simulink model "Testbench"  (R2022b)
settings: Solver=ode1  StartTime=0.0  StopTime=10.0  FixedStep=0.1  RelTol=1e-3
PreLoadFcn:
  | run("Fzg_par.m")
values from neighbouring files (symbols this model uses):
  c_alpha_H = 13400    [Fzg_Par.m]    (also in Fzg_par.m)
  c_alpha_V = 9300    [Fzg_Par.m]    (also in Fzg_par.m)
  delta_H = 0    [Fzg_Par.m]    (also in Fzg_par.m)
  delta_V = delta_L/i_L    (= 1.01419878296)    [Fzg_Par.m]    (also in Fzg_par.m = -1.01419878296)
  l_fzg = 1300/1000    (= 1.3)    [Fzg_par.m]
  l_H_fzg = 507/1000    (= 0.507)    [Fzg_Par.m]    (also in Fzg_par.m)
  l_V_fzg = 1023/1000    (= 1.023)    [Fzg_Par.m]    (also in Fzg_par.m)
  m_fzg = 241.5 + 82    (= 323.5)    [Fzg_Par.m]    (also in Fzg_par.m)
  ss_A = [-(c_alpha_V*l_V_fzg^2+c_alpha_H*l_H_fzg^2)/(J_fzg_z*v_x) (c_alpha_H*l_H_fzg-c_alpha_V*l_V_fzg)/J_fzg_z ... (first row only)    [Fzg_par.m]
  ss_B = [(c_alpha_V*l_V_fzg)/J_fzg_z -(c_alpha_H*l_H_fzg)/J_fzg_z ... (first row only)    [Fzg_par.m]
  ss_C = [1 0]    [Fzg_par.m]
  ss_D = [0 0]    [Fzg_par.m]
  v_x = 15    [Fzg_Par.m]    (also in Fzg_par.m = 10)
settings Model: LastModifiedBy=timos
settings OptimizationCC: ReuseModelBlockBuffer=on
settings RTWCC: GPUComputeCapability=5.0
settings ConfigComp: CovBoundaryAbsTol=1.0e-5

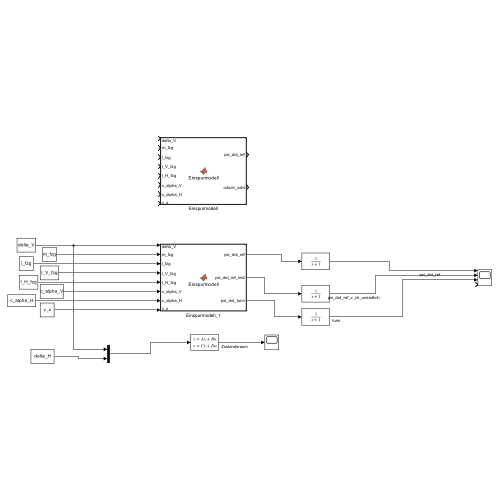
[thumbnail: Simulink's stored preview of the top-level diagram]
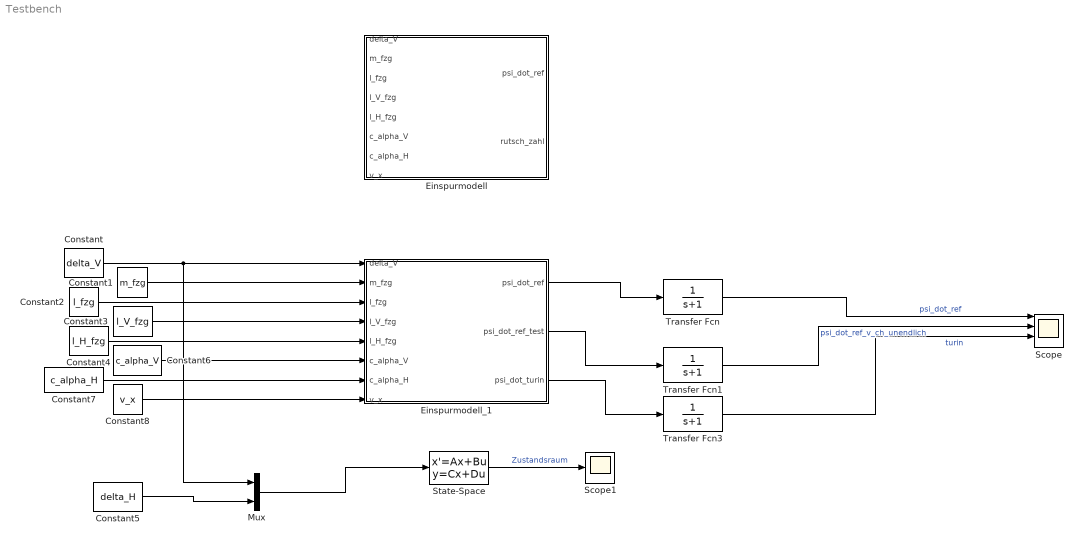
== system Testbench ==
  Constant : Constant  Value=delta_V
  Constant1 : Constant  Value=m_fzg
  Constant2 : Constant  Value=l_fzg
  Constant3 : Constant  Value=l_V_fzg
  Constant4 : Constant  Value=l_H_fzg
  Constant5 : Constant  Value=delta_H
  Constant6 : Constant  Value=c_alpha_V
  Constant7 : Constant  Value=c_alpha_H
  Constant8 : Constant  Value=v_x
  Einspurmodell : MATLAB Function  TreatAsAtomicUnit=on
  Einspurmodell_1 : MATLAB Function  TreatAsAtomicUnit=on
  Mux : Mux  Inputs=2
  Scope : Scope  NumInputPorts=4
  Scope1 : Scope
  State-Space : StateSpace  A=ss_A  B=ss_B  C=ss_C  D=ss_D  InitialCondition=0
  Transfer Fcn : TransferFcn  Denominator=[1 1]
  Transfer Fcn1 : TransferFcn  Denominator=[1 1]
  Transfer Fcn3 : TransferFcn  Denominator=[1 1]
  wires:
  Einspurmodell_1/1(psi_dot_ref) -> Transfer Fcn/1
  Constant/1 -> Mux/1, Einspurmodell_1/1(delta_V)
  Constant1/1 -> Einspurmodell_1/2(m_fzg)
  Constant2/1 -> Einspurmodell_1/3(l_fzg)
  Constant3/1 -> Einspurmodell_1/4(l_V_fzg)
  Constant4/1 -> Einspurmodell_1/5(l_H_fzg)
  Constant6/1 -> Einspurmodell_1/6(c_alpha_V)
  Constant7/1 -> Einspurmodell_1/7(c_alpha_H)
  Constant8/1 -> Einspurmodell_1/8(v_x)
  Einspurmodell_1/2(psi_dot_ref_test) -> Transfer Fcn1/1
  Transfer Fcn1/1 -> Scope/2  "psi_dot_ref_v_ch_unendlich"
  Constant5/1 -> Mux/2
  Mux/1 -> State-Space/1
  Transfer Fcn/1 -> Scope/1  "psi_dot_ref"
  Einspurmodell_1/3(psi_dot_turin) -> Transfer Fcn3/1
  Transfer Fcn3/1 -> Scope/3  "turin"
  State-Space/1 -> Scope1/1  "Zustandsraum"

== matlab function Testbench/Einspurmodell_1 ==
  data: psi_dot_ref output; delta_V input; m_fzg input; l_fzg input; l_V_fzg input; l_H_fzg input; c_alpha_V input; c_alpha_H input; v_x input; psi_dot_ref_test output; psi_dot_turin output
function [psi_dot_ref, psi_dot_ref_test, psi_dot_turin]  = Einspurmodell(delta_V, m_fzg, l_fzg, l_V_fzg, l_H_fzg, c_alpha_V, c_alpha_H, v_x)
%#codegen

% Charakteristische Geschwindigkeit zum Quadrat
square_v_ch = c_alpha_V * c_alpha_H * l_fzg / (m_fzg * ((c_alpha_H * l_H_fzg) - (c_alpha_V * l_V_fzg)));

K_turin = m_fzg/(l_fzg) * ((l_H_fzg/c_alpha_V) - (l_V_fzg/c_alpha_H));

% Soll Gierrate
psi_dot_ref = v_x * delta_V / (l_fzg * (1 + (v_x^2 / square_v_ch)));
psi_dot_ref_test = v_x * delta_V / l_fzg;
psi_dot_turin = v_x * delta_V / (l_fzg + (K_turin * v_x^2));
end

== matlab function Testbench/Einspurmodell ==
  data: psi_dot_ref output; delta_V input; m_fzg input; l_fzg input; l_V_fzg input; l_H_fzg input; c_alpha_V input; c_alpha_H input; v_x input; rutsch_zahl output
function [psi_dot_ref, rutsch_zahl]   = Einspurmodell(delta_V, m_fzg, l_fzg, l_V_fzg, l_H_fzg, c_alpha_V, c_alpha_H, v_x)
%#codegen

% Charakteristische Geschwindigkeit zum Quadrat
square_v_ch = c_alpha_V * c_alpha_H * l_fzg / (m_fzg * ((c_alpha_H * l_H_fzg) - (c_alpha_V * l_V_fzg)));

% Soll Gierrate
psi_dot_ref = v_x * delta_V / (l_fzg * (1 + (v_x^2 / square_v_ch)));

rutsch_zahl = v_x^2/square_v_ch;
end
